simulink model "pract_1"  (R2020b)
settings: Solver=VariableStepAuto  StartTime=0.0  StopTime=10.0  RelTol=1e-3
settings Model: Creator=Egor  LastModifiedBy=Egor

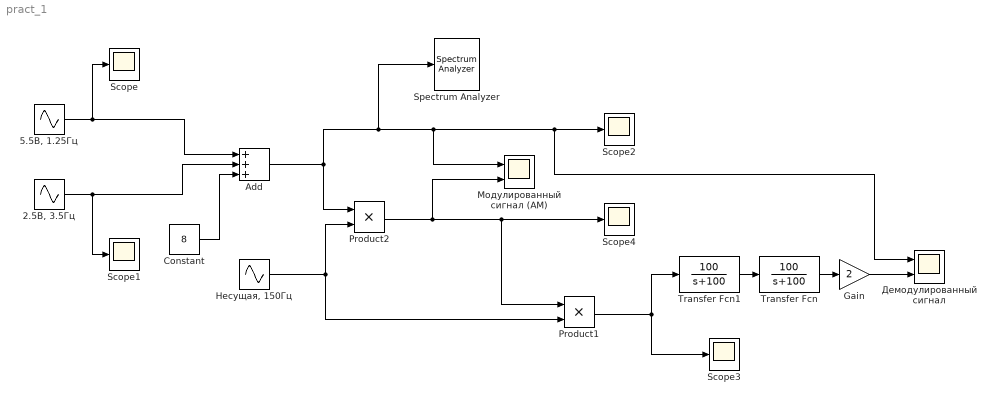
== system pract_1 ==
  "2.5В, 3.5Гц" : Sin  Amplitude=2.5  Frequency=22  SampleTime=0.001
  "5.5В, 1.25Гц" : Sin  Amplitude=5.5  Frequency=7.85  SampleTime=0.001
  Add : Sum  Inputs=+++
  Constant : Constant  Value=8
  Gain : Gain  Gain=2
  Product1 : Product
  Product2 : Product
  Scope{,1..4} (5 alike) : Scope
  Spectrum Analyzer : SpectrumAnalyzer
  Transfer Fcn : TransferFcn  Numerator=[100]  Denominator=[1 100]
  Transfer Fcn1 : TransferFcn  Numerator=[100]  Denominator=[1 100]
  Демодулированный сигнал : Scope  NumInputPorts=2
  Модулированный сигнал (АМ) : Scope  NumInputPorts=2
  "Несущая, 150Гц" : Sin  Frequency=942.5  SampleTime=0.001
  wires:
  "2.5В, 3.5Гц"/1 -> Scope1/1, Add/2
  Add/1 -> Product2/1, Модулированный сигнал (АМ)/1, Демодулированный сигнал/1, Scope2/1, Spectrum Analyzer/1
  "5.5В, 1.25Гц"/1 -> Scope/1, Add/1
  "Несущая, 150Гц"/1 -> Product2/2, Product1/2
  Product2/1 -> Scope4/1, Product1/1, Модулированный сигнал (АМ)/2
  Product1/1 -> Transfer Fcn1/1, Scope3/1
  Constant/1 -> Add/3
  Transfer Fcn/1 -> Gain/1
  Transfer Fcn1/1 -> Transfer Fcn/1
  Gain/1 -> Демодулированный сигнал/2
